simulink model "controller"  (R2023b)
settings: Solver=FixedStepAuto  StartTime=0.0  StopTime=10.0  FixedStep=1/100  RelTol=1e-3
undefined symbols (not defined in the file): MAX_TORQUE, MAX_TORQUE_REVERSE
settings Model: Creator=DAUIN-Win10  LastModifiedBy=Matteo
settings OptimizationCC: ReuseModelBlockBuffer=off
settings DebuggingCC: UnconnectedInputMsg=warning  UnconnectedOutputMsg=warning  UnconnectedLineMsg=warning
settings ModelReferenceCC: EnableRefExpFcnMdlSchedulingChecks=on
settings RTWCC: DLArmComputeVersion=19.05

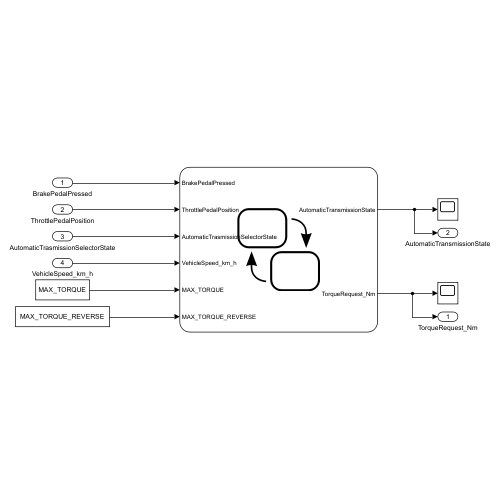
[thumbnail: Simulink's stored preview of the top-level diagram]
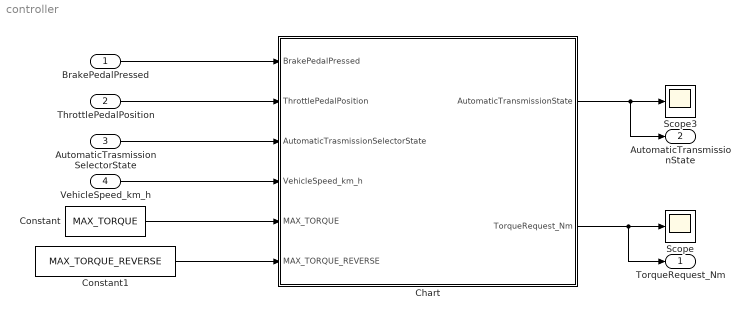
== system controller ==
  BrakePedalPressed : Inport  OutDataTypeStr=boolean
  ThrottlePedalPosition : Inport  Port=2  OutDataTypeStr=single
  AutomaticTrasmissionSelectorState : Inport  Port=3  OutDataTypeStr=Enum: TransmissionState
  VehicleSpeed_km_h : Inport  Port=4  OutDataTypeStr=single  Unit=km/h
  Chart : Stateflow chart  TreatAsAtomicUnit=on
  Constant : Constant  Value=MAX_TORQUE
  Constant1 : Constant  Value=MAX_TORQUE_REVERSE
  Scope : Scope
  Scope3 : Scope
  TorqueRequest_Nm : Outport  OutDataTypeStr=single  Unit=N*m
  AutomaticTransmissionState : Outport  Port=2  OutDataTypeStr=Enum: TransmissionState
  wires:
  BrakePedalPressed/1 -> Chart/1(BrakePedalPressed)
  ThrottlePedalPosition/1 -> Chart/2(ThrottlePedalPosition)
  AutomaticTrasmissionSelectorState/1 -> Chart/3(AutomaticTrasmissionSelectorState)
  VehicleSpeed_km_h/1 -> Chart/4(VehicleSpeed_km_h)
  Chart/2(TorqueRequest_Nm) -> TorqueRequest_Nm/1, Scope/1
  Chart/1(AutomaticTransmissionState) -> Scope3/1, AutomaticTransmissionState/1
  Constant/1 -> Chart/5(MAX_TORQUE)
  Constant1/1 -> Chart/6(MAX_TORQUE_REVERSE)

== stateflow chart controller/Chart ==
  settings: executeAtInitialization=1
  state BRAKE
    state NOMINAL_BRAKE
      entry:
      AutomaticTransmissionState=TransmissionState.Brake;
      stopping=0;
      during:
      if(ThrottlePedalPosition > 1/3)
      TorqueRequest_Nm = MAX_TORQUE * (3/2) * (ThrottlePedalPosition-1/3);
      elseif (ThrottlePedalPosition<=1/3 && VehicleSpeed_km_h>0)
      TorqueRequest_Nm = -MAX_TORQUE * (1-3*ThrottlePedalPosition);
      elseif (ThrottlePedalPosition<=1/3 && VehicleSpeed_km_h<0)
      TorqueRequest_Nm=single(0);
      stopping = 1;
      end
    state STOPPING
      entry:
      Kp = 0.5; %h/Km
      during:
      if(VehicleSpeed_km_h<0)
      TorqueRequest_Nm=Kp*MAX_TORQUE*(-VehicleSpeed_km_h);
      else
      TorqueRequest_Nm=0;
      stopping=0;
      end
    (default) -> NOMINAL_BRAKE
    NOMINAL_BRAKE -> STOPPING : [stopping==1]
    STOPPING -> NOMINAL_BRAKE : [stopping==0]
  state PARK
    entry:
    AutomaticTransmissionState=TransmissionState.Park;
    during:
    TorqueRequest_Nm = single(0);
  state DRIVE
    entry:
    AutomaticTransmissionState=TransmissionState.Drive;
    during:
    TorqueRequest_Nm = MAX_TORQUE*ThrottlePedalPosition;
  state NEUTRAL
    entry:
    AutomaticTransmissionState=TransmissionState.Neutral;
    during:
    TorqueRequest_Nm = single(0);
  state REVERSE
    entry:
    AutomaticTransmissionState=TransmissionState.Reverse;
    during:
    TorqueRequest_Nm = -MAX_TORQUE_REVERSE*ThrottlePedalPosition;
  (default) -> PARK
  NEUTRAL -> PARK [order 3] : [abs(VehicleSpeed_km_h)<5 && BrakePedalPressed==1 ...
      |  && AutomaticTrasmissionSelectorState<TransmissionState.Reverse]
  PARK -> NEUTRAL : [BrakePedalPressed==1 ...
      | && AutomaticTrasmissionSelectorState>TransmissionState.Park]
  DRIVE -> BRAKE [order 1] : [ThrottlePedalPosition>1/3 ...
      | && AutomaticTrasmissionSelectorState>TransmissionState.Drive]
  BRAKE -> DRIVE : [AutomaticTrasmissionSelectorState<TransmissionState.Brake]
  DRIVE -> NEUTRAL [order 2] : [AutomaticTrasmissionSelectorState<TransmissionState.Drive]
  NEUTRAL -> REVERSE [order 2] : [VehicleSpeed_km_h<5 && BrakePedalPressed==1 ...
      | && (AutomaticTrasmissionSelectorState<TransmissionState.Neutral ...
      | && AutomaticTrasmissionSelectorState>TransmissionState.Park)]
  NEUTRAL -> DRIVE [order 1] : [VehicleSpeed_km_h>-5 && BrakePedalPressed==1 ...
      | && AutomaticTrasmissionSelectorState>TransmissionState.Neutral]
  REVERSE -> NEUTRAL : [AutomaticTrasmissionSelectorState>TransmissionState.Reverse]
  data: BrakePedalPressed input; ThrottlePedalPosition input; AutomaticTrasmissionSelectorState input; VehicleSpeed_km_h input; AutomaticTransmissionState output; TorqueRequest_Nm output; MAX_TORQUE input; MAX_TORQUE_REVERSE input; stopping local; Kp local
